simulink model "CoolingPWM"  (R2024b)
settings: configuration reference "STM32H7_Config" (kept outside this file)
libraries: simulink x1
settings Model: DataDictionary=Master_Dictionary.sldd  EnableAccessToBaseWorkspace=off  Creator=torni  LastModifiedBy=William
settings ConfigSetRef: SourceName=STM32H7_Config

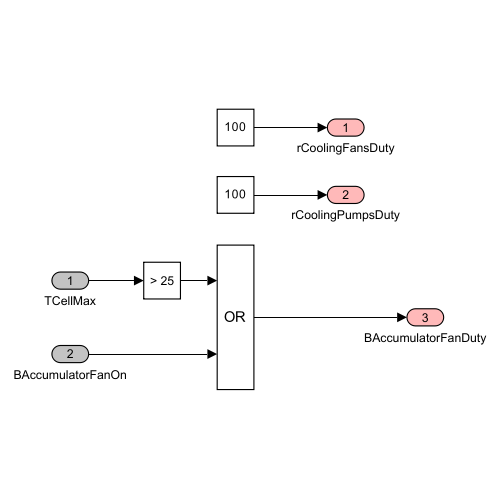
[thumbnail: Simulink's stored preview of the top-level diagram]
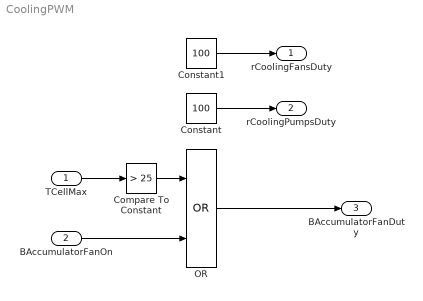
== system CoolingPWM ==
  TCellMax : Inport  OutDataTypeStr=double
  BAccumulatorFanOn : Inport  Port=2  OutDataTypeStr=boolean
  Compare To Constant : simulink/Logic and Bit Operations/Compare To Constant  relop=>  const=25  OutDataTypeStr=boolean
  Constant : Constant  Value=100
  Constant1 : Constant  Value=100
  OR : Logic  Operator=OR  AllPortsSameDT=off  OutDataTypeStr=boolean
  rCoolingFansDuty : Outport  OutDataTypeStr=double  VectorParamsAs1DForOutWhenUnconnected=off
  rCoolingPumpsDuty : Outport  Port=2  OutDataTypeStr=double  VectorParamsAs1DForOutWhenUnconnected=off
  BAccumulatorFanDuty : Outport  Port=3  OutDataTypeStr=boolean  VectorParamsAs1DForOutWhenUnconnected=off
  wires:
  Constant1/1 -> rCoolingFansDuty/1
  Constant/1 -> rCoolingPumpsDuty/1
  TCellMax/1 -> Compare To Constant/1
  Compare To Constant/1 -> OR/1
  BAccumulatorFanOn/1 -> OR/2
  OR/1 -> BAccumulatorFanDuty/1
